simulink model "ENV_scheduled"  (R2024b)
settings: Solver=FixedStepDiscrete  StartTime=0.0  StopTime=10.0  FixedStep=0.001  RelTol=1e-3
libraries: stm32blockslib x54, canmsglib x29, simulink x7, stm32f4xxblockslib x1
(part 1 of 5)
settings Model: DataDictionary=Master_Dictionary.sldd  EnableAccessToBaseWorkspace=off  STM32="{\"SPIControllerTransfer\":[{\"ID\":\"ENV:1198\"},{\"ID\":\"ENV:1199\"},{\"ID\":\"ENV:1337\"},{\"ID\":\"ENV:1338\"},{\"ID\":\"ENV:1339\"},{\"ID\":\"ENV:1340\"},{\"ID\":\"ENV:1341\"},{\"ID\":\"ENV:1354\"},{\"ID\":\"ENV:1361\"},{\"ID\":\"ENV:1368\"},{\"ID\":\"ENV:1375\"},{\"ID\":\"ENV:1394\"},{\"ID\":\"ENV:1413\"},{\"ID\":\"ENV:1469\"},{\"ID\":\"ENV:2306\"},{\"ID\":\"ENV:2307\"},{\"ID\":\"ENV:2328\"},{\"ID\":\"ENV:2329\"},{\"ID\":\"ENV:2371\"},{\"ID\":\"ENV:2372\"},{\"ID\":\"ENV:2383\"},{\"ID\":\"ENV:2384\"},{\"ID\":\"ENV:2395\"},{\"ID\":\"ENV:2396\"},{\"ID\":\"ENV:2407\"},{\"ID\":\"ENV:2408\"},{\"ID\":\"ENV:2419\"},{\"ID\":\"ENV:2420\"},{\"ID\":\"ENV:2431\"},{\"ID\":\"ENV:2432\"},{\"ID\":\"ENV:2443\"},{\"ID\":\"ENV:2444\"},{\"ID\":\"ENV:2455\"},{\"ID\":\"ENV:2456\"},{\"ID\":\"ENV:2467\"},{\"ID\":\"ENV:2468\"},{\"ID\":\"ENV:2479\"},{\"ID\":\"ENV:2480\"},{\"ID\":\"ENV:2491\"},{\"ID\":\"ENV:2492\"},{\"ID\":\"ENV:2503\"},{\"ID\":\"ENV:2504\"},{\"ID\":\"ENV:2515\"},{\"ID\":\"ENV:2516\"},{\"ID\":\"ENV:2527\"},{\"ID\":\"ENV:2528\"},{\"ID\":\"ENV:2539\"},{\"ID\":\"ENV:2540\"},{\"ID\":\"ENV:2551\"},{\"ID\":\"ENV:2552\"},{\"ID\":\"ENV:2563\"},{\"ID\":\"ENV:2564\"},{\"ID\":\"ENV:2575\"},{\"ID\":\"ENV:2576\"}],\"DigitalPortRead\":{\"ID\":\"ENV:1217\"}}"  Creator=oxbro  LastModifiedBy=oxbro
settings SolverCC: AlgebraicLoopSolver=TrustRegion
settings DataIOCC: ReturnWorkspaceOutputs=off
settings OptimizationCC: DefaultParameterBehavior=Inlined  OptimizeBlockIOStorage=off  BufferReuse=off  ReuseModelBlockBuffer=off  GlobalBufferReuse=off  ExpressionFolding=off  EnableMemcpy=off  PassReuseOutputArgsAs=Individual arguments  LocalBlockOutputs=off  ZeroExternalMemoryAtStartup=off  ZeroInternalMemoryAtStartup=off  MaxStackSize=8192  OptimizeDataStoreBuffers=off  BusAssignmentInplaceUpdate=off  OptimizationLevel=level0  OptimizationCustomize=off  EfficientTunableParamExpr=on
settings DebuggingCC: ParameterOverflowMsg=warning  ParameterTunabilityLossMsg=error  UnconnectedInputMsg=warning  UnconnectedOutputMsg=warning  UnconnectedLineMsg=warning  ArithmeticOperatorsInVariantConditions=warning
settings HardwareCC: ProdBitPerPointer=32  ProdBitPerSizeT=32  ProdBitPerPtrDiffT=32  ProdLargestAtomicInteger=Long  ProdLargestAtomicFloat=Double  ProdWordSize=32  ProdLongLongMode=on  ProdHWDeviceType=ARM Compatible->ARM Cortex-M
settings ModelReferenceCC: EnableRefExpFcnMdlSchedulingChecks=on
settings SFSimCC: MATLABDynamicMemAlloc=off  CustomCodeUndefinedFunction=UseInterfaceOnly
settings RTWCC: Description=Embedded Coder  SystemTargetFile=ert.tlc  HardwareBoard=STM32H7xx Based (Single-core)  TemplateMakefile=ert_default_tmf  Toolchain=GNU Tools for ARM Embedded Processors  GPUComputeCapability=3.5
settings CodeAppCC: ForceParamTrailComments=on  IgnoreCustomStorageClasses=off  MaxIdLength=45  OperatorAnnotations=on  SimulinkDataObjDesc=on  SFDataObjDesc=on  InsertBlockDesc=on
settings ERTTargetCC: TargetLangStandard=C99 (ISO)  CodeReplacementLibrary=ARM Cortex-M  ExtModeTransport=3  ExtModeStaticAlloc=on  ExtModeStaticAllocSize=2048  ExtModeMexFile=ext_xcp  ExtModeIntrfLevel=Level2 - Open

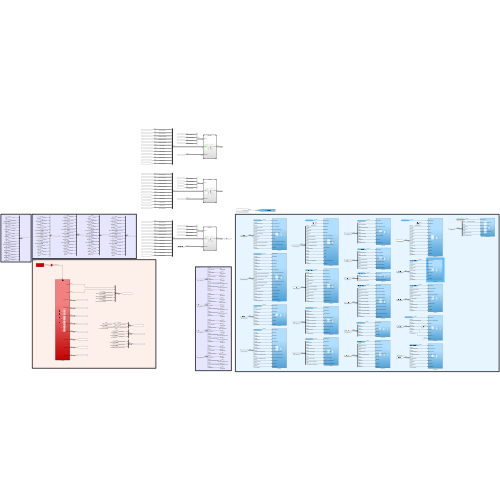
[thumbnail: Simulink's stored preview of the top-level diagram]
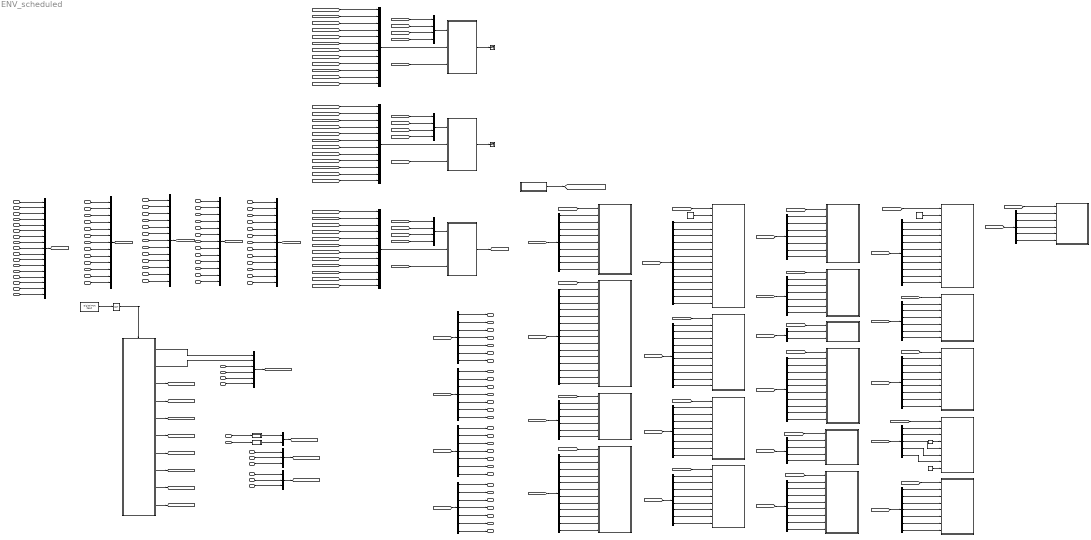
== system ENV_scheduled ==
  note: CAN3
  note: CAN 1&2
  note: CAN3
  note: CAN4
  note: CAN1&2
  nMotorRL : Inport
  BInvDCOnRLIn : Inport  Port=2
  BInvErrorRL : Inport  Port=3
  BInvOnRLIn : Inport  Port=4
  BInvDCQuitInvOnRL : Inport  Port=5
  BInvQuitInvOnRL : Inport  Port=6
  BInvSysReadyRL : Inport  Port=7
  BInvWarnRL : Inport  Port=8
  MMotorMeasuredRL : Inport  Port=9
  NInvDTCRL : Inport  Port=10
  TMotorRL : Inport  Port=11
  VDCInvRL : Inport  Port=12
  TInvRL : Inport  Port=13
  nMotorRR : Inport  Port=14
  BInvDCOnRRIn : Inport  Port=15
  BInvErrorRR : Inport  Port=16
  BInvOnRRIn : Inport  Port=17
  BInvDCQuitInvOnRR : Inport  Port=18
  BInvQuitInvOnRR : Inport  Port=19
  BInvSysReadyRR : Inport  Port=20
  BInvWarnRR : Inport  Port=21
  MMotorMeasuredRR : Inport  Port=22
  NInvDTCRR : Inport  Port=23
  TMotorRR : Inport  Port=24
  VDCInvRR : Inport  Port=25
  TInvRR : Inport  Port=26
  nMotorFL : Inport  Port=27
  BInvDCOnFLIn : Inport  Port=28
  BInvErrorFL : Inport  Port=29
  BInvOnFLIn : Inport  Port=30
  BInvDCQuitInvOnFL : Inport  Port=31
  BInvQuitInvOnFL : Inport  Port=32
  BInvSysReadyFL : Inport  Port=33
  BInvWarnFL : Inport  Port=34
  MMotorMeasuredFL : Inport  Port=35
  NInvDTCFL : Inport  Port=36
  TMotorFL : Inport  Port=37
  VDCInvFL : Inport  Port=38
  TInvFL : Inport  Port=39
  nMotorFR : Inport  Port=40
  BInvDCOnFR : Inport  Port=41
  BInvErrorFR : Inport  Port=42
  BInvOnFR : Inport  Port=43
  BInvDCQuitInvOnFR : Inport  Port=44
  BInvQuitInvOnFR : Inport  Port=45
  BInvSysReadyFR : Inport  Port=46
  BInvWarnFR : Inport  Port=47
  MMotorMeasuredFR : Inport  Port=48
  NInvDTCFR : Inport  Port=49
  TMotorFR : Inport  Port=50
  VDCInvFR : Inport  Port=51
  TInvFR : Inport  Port=52
  IIVTS : Inport  Port=53
  IBMSHallEffect : Inport  Port=54
  VDCAccumulator : Inport  Port=55
  TCellMin : Inport  Port=56
  VCellAverage : Inport  Port=57
  VCellMax : Inport  Port=58
  TCellMax : Inport  Port=59
  NBMSDLC : Inport  Port=60
  VCellMin : Inport  Port=61
  RCellAverage : Inport  Port=62
  BBalancingActive : Inport  Port=63
  BBMSP0A0C : Inport  Port=64  OutDataTypeStr=double
  BBMSP0A0E : Inport  Port=65
  BBMSP0A10 : Inport  Port=66
  BBMSP0A80 : Inport  Port=67
  BBMSP0AC0 : Inport  Port=68
  BBMSP0AFA : Inport  Port=69
  vLateralOXTSIMU : Inport  Port=70
  vLongitudinalOXTSIMU : Inport  Port=71
  gLateralOXTS : Inport  Port=72
  gLongitudinalOXTS : Inport  Port=73
  gVerticalOXTS : Inport  Port=74
  nPitchRateOXTSIMU : Inport  Port=75
  nRollRateOXTSIMU : Inport  Port=76
  nYawRateOXTSIMU : Inport  Port=77
  VDamperPotentiometerFL : Inport  Port=78
  VDamperPotentiometerFR : Inport  Port=79
  VDamperPotentiometerRR : Inport  Port=80
  VDamperPotentiometerRL : Inport  Port=81
  Bus Creator1 : BusCreator  Inputs=6  OutDataTypeStr=Bus: DDU7_Analoge_1
  Bus Creator13 : BusCreator  Inputs=12  OutDataTypeStr=Bus: CAN3Bus
  Bus Creator14 : BusCreator  Inputs=13  OutDataTypeStr=Bus: InverterFLCANBus
  Bus Creator15 : BusCreator  Inputs=13  OutDataTypeStr=Bus: InverterFRCANBus
  Bus Creator16 : BusCreator  Inputs=12  OutDataTypeStr=Bus: CAN3Bus
  Bus Creator17 : BusCreator  Inputs=13  OutDataTypeStr=Bus: InverterRLCANBus
  Bus Creator18 : BusCreator  Inputs=17  OutDataTypeStr=Bus: CAN4Bus
  Bus Creator19 : BusCreator  Inputs=13  OutDataTypeStr=Bus: InverterRRCANBus
  Bus Creator20 : BusCreator  Inputs=12  OutDataTypeStr=Bus: CAN3Bus
  Bus Creator6 : BusCreator  Inputs=3  OutDataTypeStr=Bus: OXTSDataFrame1544
  Bus Creator7 : BusCreator  Inputs=3  OutDataTypeStr=Bus: OXTSDataFrame1541
  Bus Creator8 : BusCreator  Inputs=2  OutDataTypeStr=Bus: OXTSDataFrame1540
  Bus Selector : BusSelector  OutputSignals=SystemsBus.BEncoderErrorFront,SystemsBus.BEncoderErrorRear,SystemsBus.BSpinningModelActivated,TorqueControlBus.BTorqueVectoringOK,TorqueControlBus.MTotalFinal,SystemsBus.PActual,TorqueControlBus.PPowerControllerProportionalTerm,TorqueControlBus.PPowerControllerIntegralTerm,SystemsBus.vChassis
  Bus Selector1 : BusSelector  OutputSignals=BMSSignalsBus.BBMSP0A80,BMSSignalsBus.BBMSP0AC0,BMSSignalsBus.BBMSP0AFA,SystemsBus.PDischarge,LimitationsBus.rDischargeDerate,LimitationsBus.rHighCellTemperatureDischargeDerate,LimitationsBus.rHighCellTemperatureRegenDerate,LimitationsBus.rInvTemperatureDerate,LimitationsBus.rLowCellVoltageDischargeDerate,LimitationsBus.rMotorTemperatureDerate,LimitationsBus.rRegenDerate,LimitationsBus.rSOCDischargeDerate,LimitationsBus.rSOCRegenDerate,TorqueControlBus.rSOCTargetError,LimitationsBus.rSpeedRegenDerate
  Bus Selector10 : BusSelector  OutputSignals=SensorSignalsBus.VDamperPotentiometerFL,SensorSignalsBus.VDamperPotentiometerFR
  Bus Selector11 : BusSelector  OutputSignals=TorqueControlBus.MTotalEMSRequested,LimitationsBus.rInvTemperatureDerateFL,LimitationsBus.rInvTemperatureDerateFR,LimitationsBus.rInvTemperatureDerateRL,LimitationsBus.rInvTemperatureDerateRR,LimitationsBus.rMotorTemperatureDerateFL,LimitationsBus.rMotorTemperatureDerateFR,LimitationsBus.rMotorTemperatureDerateRL,LimitationsBus.rMotorTemperatureDerateRR,SystemsBus.rThrottlePedal
  Bus Selector12 : BusSelector  OutputSignals=InverterSignalsBus.InverterFLSignalsBus.nMotorFL,InverterSignalsBus.InverterFRSignalsBus.nMotorFR,InverterSignalsBus.InverterRLSignalsBus.nMotorRL,InverterSignalsBus.InverterRRSignalsBus.nMotorRR
  Bus Selector13 : BusSelector  OutputSignals=LimitationsBus.BDischargeAllowed,SystemsBus.BEMS1000mPoint,SystemsBus.BEMS995mPoint,TorqueControlBus.MDriverDischargeRequested,TorqueControlBus.MFLFinal,TorqueControlBus.MFRFinal,TorqueControlBus.MRLFinal,TorqueControlBus.MRRFinal
  Bus Selector14 : BusSelector  OutputSignals=InverterSignalsBus.InverterFLSignalsBus.TInvFL,InverterSignalsBus.InverterFRSignalsBus.TInvFR,SystemsBus.TInvMax,InverterSignalsBus.InverterRLSignalsBus.TInvRL,InverterSignalsBus.InverterRRSignalsBus.TInvRR,InverterSignalsBus.InverterFLSignalsBus.TMotorFL,InverterSignalsBus.InverterFRSignalsBus.TMotorFR,SystemsBus.TMotorMax,InverterSignalsBus.InverterRLSignalsBus.TMotorRL,InverterSignalsBus.InverterRRSignalsBus.TMotorRR
  Bus Selector15 : BusSelector  OutputSignals=InverterSignalsBus.InverterFLSignalsBus.NInvDTCFL,InverterSignalsBus.InverterFRSignalsBus.NInvDTCFR,InverterSignalsBus.InverterRLSignalsBus.NInvDTCRL,InverterSignalsBus.InverterRRSignalsBus.NInvDTCRR,BMSSignalsBus.TCellMax,BMSSignalsBus.VCellDelta
  Bus Selector16 : BusSelector  OutputSignals=SystemsBus.BAccumulatorFanOn,SystemsBus.BEMSActivated,SystemsBus.BTractionControlActivated,BMSSignalsBus.IBMSHallEffect,BMSSignalsBus.IIVTS,TorqueControlBus.MTotalRequested,BMSSignalsBus.VDCAccumulator,InverterSignalsBus.InverterRLSignalsBus.VDCInvRL
  Bus Selector17 : BusSelector  OutputSignals=SystemsBus.NTractionControlKpSelector,BMSSignalsBus.TCellMin,BMSSignalsBus.VCellMax,BMSSignalsBus.VCellMin,SensorSignalsBus.VLVSystem
  Bus Selector18 : BusSelector  OutputSignals=TorqueControlBus.PDischargeLimited,SystemsBus.aSteeringAngle,TorqueControlBus.nYawRateErrorActual,SystemsBus.rRegenPaddle,TorqueControlBus.rSplitRear,SystemsBus.tAppsTimer,SystemsBus.tPedalOverlap
  Bus Selector2 : BusSelector  OutputSignals=TorqueControlBus.rSOETargetError,SystemsBus.sEMS1000m,WheelSpeedsBus.vWheelFL,WheelSpeedsBus.vWheelFR,WheelSpeedsBus.vWheelRL,WheelSpeedsBus.vWheelRR
  Bus Selector20 : BusSelector  OutputSignals=StateflowBus.BInvDCOnRL,StateflowBus.BInvEnableRL,StateflowBus.BInvErrorResetRL,StateflowBus.BInvOnRL,StateflowBus.MTorqueLimitNegativeRL,StateflowBus.MTorqueLimitPositiveRL,TorqueControlBus.MRLFinal
  Bus Selector21 : BusSelector  OutputSignals=StateflowBus.BInvDCOnFL,StateflowBus.BInvEnableFL,StateflowBus.BInvErrorResetFL,StateflowBus.BInvOnFL,StateflowBus.MTorqueLimitNegativeFL,StateflowBus.MTorqueLimitPositiveFL,TorqueControlBus.MFLFinal
  Bus Selector22 : BusSelector  OutputSignals=StateflowBus.BInvDCOnRR,StateflowBus.BInvEnableRR,StateflowBus.BInvErrorResetRR,StateflowBus.BInvOnRR,StateflowBus.MTorqueLimitNegativeRR,StateflowBus.MTorqueLimitPositiveRR,TorqueControlBus.MRRFinal
  Bus Selector23 : BusSelector  OutputSignals=StateflowBus.BInvDCOnFR,StateflowBus.BInvEnableFR,StateflowBus.BInvErrorResetFR,StateflowBus.BInvOnFR,StateflowBus.MTorqueLimitNegativeFR,StateflowBus.MTorqueLimitPositiveFR,TorqueControlBus.MFRFinal
  Bus Selector27 : BusSelector  OutputSignals=SystemsBus.BAccumulatorFanOn,SystemsBus.BBrakeLight,SystemsBus.BInvLVOn,StateflowBus.BReadyToDriveBuzzer,SystemsBus.BAccumulatorFanDuty
  Bus Selector3 : BusSelector  OutputSignals=SystemsBus.BAppsOK,SystemsBus.BBrakeError,SystemsBus.BBrakeOn,SystemsBus.BPedalOverlap,SystemsBus.BRegenOn,SystemsBus.BThrottleError,SystemsBus.BTorqueVectoringActivated,TorqueControlBus.MPowerControllerRequested,TorqueControlBus.PPowerControllerRequested,SystemsBus.rThrottlePedal,SystemsBus.tBrakeError,SystemsBus.tThrottleError
  Bus Selector4 : BusSelector  OutputSignals=StateflowBus.BReadyToDrive,TorqueControlBus.NABSMultiplierRL,TorqueControlBus.NABSMultiplierRR,SystemsBus.NThrottleMap,TorqueControlBus.NTractionControlMultiplierRL,TorqueControlBus.NTractionControlMultiplierRR,TorqueControlBus.rSlipRatioFLActual,TorqueControlBus.rSlipRatioFRActual,TorqueControlBus.rSlipRatioRLActual,TorqueControlBus.rSlipRatioRRActual
  Bus Selector5 : BusSelector  OutputSignals=BMSSignalsBus.NBMSDLC,StateflowBus.NBMSState,StateflowBus.NInvState,SystemsBus.NModeNumberDisplay5,SystemsBus.NModeNumberDisplay6,SystemsBus.NPowerControllerKpSelector,SystemsBus.NTorqueSplitSpeedSelector,SystemsBus.PEngineBraking,SystemsBus.PRegen,SystemsBus.rSOC,SystemsBus.rSOE,SystemsBus.rTorqueVectoringMultiplier,SystemsBus.sChassis
  Bus Selector6 : BusSelector  OutputSignals=BMSSignalsBus.BBMSP0A0C,BMSSignalsBus.BBalancingActive,TorqueControlBus.MTractionControlFLTotal,TorqueControlBus.MTractionControlFRTotal,TorqueControlBus.MTractionControlRLTotal,TorqueControlBus.MTractionControlRRTotal,TorqueControlBus.NABSMultiplierFL,TorqueControlBus.NABSMultiplierFR
  Bus Selector7 : BusSelector  OutputSignals=BMSSignalsBus.BBMSP0A0E,BMSSignalsBus.BBMSP0A10,TorqueControlBus.MTorqueVectoringFL,TorqueControlBus.MTorqueVectoringFR,TorqueControlBus.MTorqueVectoringRL,TorqueControlBus.MTorqueVectoringRR,TorqueControlBus.NTractionControlMultiplierFL,TorqueControlBus.NTractionControlMultiplierFR
  Bus Selector8 : BusSelector  OutputSignals=TorqueControlBus.MDischargeLimited,TorqueControlBus.MDriverRegenRequested,TorqueControlBus.MRegenLimited,TorqueControlBus.MSpinningModelFL,TorqueControlBus.MSpinningModelFR,StateflowBus.NCarState,TorqueControlBus.rSlipRatioOptimal
  Bus Selector9 : BusSelector  OutputSignals=TorqueControlBus.MSpinningModelRL,TorqueControlBus.MSpinningModelRR,TorqueControlBus.MTorqueDistributionFL,TorqueControlBus.MTorqueDistributionFR,TorqueControlBus.MTorqueDistributionRL,TorqueControlBus.MTorqueDistributionRR
  CAN Rx : Subsystem  TreatAsAtomicUnit=on
  CAN Tx : Subsystem
  CAN Tx1 : Subsystem
  CAN Tx10 : Subsystem
  CAN Tx11 : Subsystem
  CAN Tx12 : Subsystem
  CAN Tx13 : Subsystem
  CAN Tx14 : Subsystem
  CAN Tx15 : Subsystem
  CAN Tx16 : Subsystem
  CAN Tx17 : Subsystem
  CAN Tx18 : Subsystem
  CAN Tx19 : Subsystem
  CAN Tx2 : Subsystem
  CAN Tx3 : Subsystem
  CAN Tx4 : Subsystem
  CAN Tx5 : Subsystem
  CAN Tx6 : Subsystem
  CAN Tx7 : Subsystem
  CAN Tx8 : Subsystem
  CAN Tx9 : Subsystem
  CAN1_2Bus : BusCreator  Inputs=4  OutDataTypeStr=Bus: CAN1_2Bus
  CAN1_2Bus1 : BusCreator  Inputs=4  OutDataTypeStr=Bus: CAN1_2Bus
  CAN1_2Bus2 : BusCreator  Inputs=4  OutDataTypeStr=Bus: CAN1_2Bus
  Constant : Constant  Value=92
  Constant1 : Constant  Value=92
  Digital Port Read1 : stm32f4xxblockslib/Digital Port Read  PortName=GPIOB  PinNumber=5  ReadOperation=on  IOAsArray=off  SampleTime=-1  EnableSimPort=off  hoistedMaskSrc=ECSoC/ECSimCodegen/Digital Port Read
      settings: LibrarySourceBlock=stm32f2xxblockslib/Digital Port Read
  Model : ModelReference  ModelNameDialog=MASTER.slx  SimulationMode=Normal  ModelReferenceVersion=13.13
  Model1 : ModelReference  ModelNameDialog=MASTER.slx  SimulationMode=Normal  ModelReferenceVersion=13.13
  Model2 : ModelReference  ModelNameDialog=MASTER.slx  SimulationMode=Normal  ModelReferenceVersion=13.13
  Multiplexer1? : simulink/Sources/Counter Limited  uplimit=1  tsamp=5
  Multiplexer? : simulink/Sources/Counter Limited  uplimit=1  tsamp=5
  NOT4 : Logic  Operator=NOT  IconShape=distinctive  AllPortsSameDT=off  OutDataTypeStr=boolean
  Subsystem : Subsystem
  Terminator : Terminator
  Terminator1 : Terminator
  gLat : Subsystem
  gLong : Subsystem
  BInvDCOnRL : Outport  VectorParamsAs1DForOutWhenUnconnected=off
  BInvEnableRL : Outport  Port=2  VectorParamsAs1DForOutWhenUnconnected=off
  BInvErrorResetRL : Outport  Port=3  VectorParamsAs1DForOutWhenUnconnected=off
  BInvOnRL : Outport  Port=4  VectorParamsAs1DForOutWhenUnconnected=off
  MTorqueLimitNegativeRL : Outport  Port=5  VectorParamsAs1DForOutWhenUnconnected=off
  MTorqueLimitPositiveRL : Outport  Port=6  VectorParamsAs1DForOutWhenUnconnected=off
  MInvRLFinal : Outport  Port=7  VectorParamsAs1DForOutWhenUnconnected=off
  BInvDCOnFL : Outport  Port=8  VectorParamsAs1DForOutWhenUnconnected=off
  BInvEnableFL : Outport  Port=9  VectorParamsAs1DForOutWhenUnconnected=off
  BInvErrorResetFL : Outport  Port=10  VectorParamsAs1DForOutWhenUnconnected=off
  BInvOnFL : Outport  Port=11  VectorParamsAs1DForOutWhenUnconnected=off
  MTorqueLimitNegativeFL : Outport  Port=12  VectorParamsAs1DForOutWhenUnconnected=off
  MTorqueLimitPositiveFL : Outport  Port=13  VectorParamsAs1DForOutWhenUnconnected=off
  MInvFLFinal : Outport  Port=14  VectorParamsAs1DForOutWhenUnconnected=off
  BInvDCOnRR : Outport  Port=15  VectorParamsAs1DForOutWhenUnconnected=off
  BInvEnableRR : Outport  Port=16  VectorParamsAs1DForOutWhenUnconnected=off
  BInvErrorResetRR : Outport  Port=17  VectorParamsAs1DForOutWhenUnconnected=off
  BInvOnRR : Outport  Port=18  VectorParamsAs1DForOutWhenUnconnected=off
  MTorqueLimitNegativeRR : Outport  Port=19  VectorParamsAs1DForOutWhenUnconnected=off
  MTorqueLimitPositiveRR : Outport  Port=20  VectorParamsAs1DForOutWhenUnconnected=off
  MInvRRFinal : Outport  Port=21  VectorParamsAs1DForOutWhenUnconnected=off
  "BInvDCOnFR " : Outport  Port=22  VectorParamsAs1DForOutWhenUnconnected=off
  BInvEnableFR : Outport  Port=23  VectorParamsAs1DForOutWhenUnconnected=off
  BInvErrorResetFR : Outport  Port=24  VectorParamsAs1DForOutWhenUnconnected=off
  "BInvOnFR " : Outport  Port=25  VectorParamsAs1DForOutWhenUnconnected=off
  MTorqueLimitNegativeFR : Outport  Port=26  VectorParamsAs1DForOutWhenUnconnected=off
  MTorqueLimitPositiveFR : Outport  Port=27  VectorParamsAs1DForOutWhenUnconnected=off
  MInvFRFinal : Outport  Port=28  VectorParamsAs1DForOutWhenUnconnected=off
  wires:
  nMotorRL/1 -> Bus Creator17/1  "nMotorRL"
  BInvDCOnRLIn/1 -> Bus Creator17/2  "BInvDCOnRL"
  BInvErrorRL/1 -> Bus Creator17/3  "BInvErrorRL"
  BInvOnRLIn/1 -> Bus Creator17/4  "BInvOnRL"
  BInvDCQuitInvOnRL/1 -> Bus Creator17/5  "BInvDCQuitInvOnRL"
  BInvSysReadyRL/1 -> Bus Creator17/7  "BInvSysReadyRL"
  BInvWarnRL/1 -> Bus Creator17/8  "BInvWarnRL"
  MMotorMeasuredRL/1 -> Bus Creator17/9  "MMotorMeasuredRL"
  NInvDTCRL/1 -> Bus Creator17/10  "NInvDTCRL"
  TMotorRL/1 -> Bus Creator17/11  "TMotorRL"
  VDCInvRL/1 -> Bus Creator17/12  "VDCInvRL"
  MMotorMeasuredRR/1 -> Bus Creator19/9  "MMotorMeasuredRR"
  BInvSysReadyRR/1 -> Bus Creator19/7  "BInvSysReadyRR"
  TMotorRR/1 -> Bus Creator19/11  "TMotorRR"
  BInvErrorRR/1 -> Bus Creator19/3  "BInvErrorRR"
  nMotorRR/1 -> Bus Creator19/1  "nMotorRR"
  BInvDCQuitInvOnRR/1 -> Bus Creator19/5  "BInvDCQuitInvOnRR"
  BInvDCOnRRIn/1 -> Bus Creator19/2  "BInvDCOnRR"
  BInvWarnRR/1 -> Bus Creator19/8  "BInvWarnRR"
  NInvDTCRR/1 -> Bus Creator19/10  "NInvDTCRR"
  VDCInvRR/1 -> Bus Creator19/12  "VDCInvRR"
  BInvOnRRIn/1 -> Bus Creator19/4  "BInvOnRR"
  BInvOnFLIn/1 -> Bus Creator14/4  "BInvOnFL"
  VDCInvFL/1 -> Bus Creator14/12  "VDCInvFL"
  BInvWarnFL/1 -> Bus Creator14/8  "BInvWarnFL"
  BInvDCQuitInvOnFL/1 -> Bus Creator14/5  "BInvDCQuitInvOnFL"
  NInvDTCFL/1 -> Bus Creator14/10  "NInvDTCFL"
  BInvErrorFL/1 -> Bus Creator14/3  "BInvErrorFL"
  BInvDCOnFLIn/1 -> Bus Creator14/2  "BInvDCOnFL"
  TMotorFL/1 -> Bus Creator14/11  "TMotorFL"
  nMotorFL/1 -> Bus Creator14/1  "nMotorFL"
  BInvSysReadyFL/1 -> Bus Creator14/7  "BInvSysReadyFL"
  MMotorMeasuredFL/1 -> Bus Creator14/9  "MMotorMeasuredFL"
  BInvDCOnFR/1 -> Bus Creator15/2  "BInvDCOnFR"
  BInvErrorFR/1 -> Bus Creator15/3  "BInvErrorFR"
  MMotorMeasuredFR/1 -> Bus Creator15/9  "MMotorMeasuredFR"
  BInvSysReadyFR/1 -> Bus Creator15/7  "BInvSysReadyFR"
  nMotorFR/1 -> Bus Creator15/1  "nMotorFR"
  TMotorFR/1 -> Bus Creator15/11  "TMotorFR"
  NInvDTCFR/1 -> Bus Creator15/10  "NInvDTCFR"
  VDCInvFR/1 -> Bus Creator15/12  "VDCInvFR"
  BInvDCQuitInvOnFR/1 -> Bus Creator15/5  "BInvDCQuitInvOnFR"
  BInvWarnFR/1 -> Bus Creator15/8  "BInvWarnFR"
  BInvOnFR/1 -> Bus Creator15/4  "BInvOnFR"
  Bus Creator17/1 -> [InverterRLBus]
  Bus Creator14/1 -> [InverterFLBus]
  Bus Creator15/1 -> [InverterFRBus]
  IIVTS/1 -> Bus Creator18/1  "IIVTS"
  TCellMin/1 -> Bus Creator18/4  "TCellMin"
  RCellAverage/1 -> Bus Creator18/10  "RCellAverage"
  TCellMax/1 -> Bus Creator18/7  "TCellMax"
  BBMSP0A80/1 -> Bus Creator18/15  "BBMSP0A80"
  IBMSHallEffect/1 -> Bus Creator18/2  "IBMSHallEffect"
  VDCAccumulator/1 -> Bus Creator18/3  "VDCAccumulator"
  VCellAverage/1 -> Bus Creator18/5  "VCellAverage"
  NBMSDLC/1 -> Bus Creator18/8  "NBMSDLC"
  VCellMin/1 -> Bus Creator18/9  "VCellMin"
  VCellMax/1 -> Bus Creator18/6  "VCellMax"
  BBalancingActive/1 -> Bus Creator18/11  "BBalancingActive"
  BBMSP0A0C/1 -> Bus Creator18/12  "BBMSP0A0C"
  BBMSP0A0E/1 -> Bus Creator18/13  "BBMSP0A0E"
  BBMSP0A10/1 -> Bus Creator18/14  "BBMSP0A10"
  BBMSP0AC0/1 -> Bus Creator18/16  "BBMSP0AC0"
  BBMSP0AFA/1 -> Bus Creator18/17  "BBMSP0AFA"
  Bus Creator18/1 -> [BMSCAN]
  Bus Creator1/1 -> [DDU7_Analoge_1]
  Bus Creator8/1 -> [OXTSDataFrame1540]
  gLateralOXTS/1 -> Bus Creator7/1  "gLateralOXTS"
  gLongitudinalOXTS/1 -> Bus Creator7/2  "gLongitudinalOXTS"
  gVerticalOXTS/1 -> Bus Creator7/3  "gVerticalOXTS"
  Bus Creator7/1 -> [OXTSDataFrame1541]
  nPitchRateOXTSIMU/1 -> Bus Creator6/1  "nPitchRateOXTSIMU"
  nRollRateOXTSIMU/1 -> Bus Creator6/2  "nRollRateOXTSIMU"
  nYawRateOXTSIMU/1 -> Bus Creator6/3  "nYawRateOXTSIMU"
  Bus Creator6/1 -> [OXTSDataFrame1544]
  CAN1_2Bus/1 -> Model/1
  [BMSCAN] -> Model/3
  [DDU7_Analoge_1] -> Bus Creator13/1  "DDU7_Analoge_1"
  [DDU7_Analoge_2] -> Bus Creator13/2  "DDU7_Analoge_2"
  [OXTSDataFrame1540] -> Bus Creator13/3  "OXTSDataFrame1540"
  [OXTSDataFrame1541] -> Bus Creator13/4  "OXTSDataFrame1541"
  [OXTSDataFrame1544] -> Bus Creator13/5  "OXTSDataFrame1544"
  [PDM_Status_1] -> Bus Creator13/6  "PDM_Status_1"
  [PDM_Status_2] -> Bus Creator13/7  "PDM_Status_2"
  [PDM_Status_3] -> Bus Creator13/8  "PDM_Status_3"
  [PDM_Analog_1] -> Bus Creator13/9  "PDM_Analoge_1"
  [PDM_Analoge_2] -> Bus Creator13/10  "PDM_Analoge_2"
  [PDM_Analoge_3] -> Bus Creator13/11  "PDM_Analoge_3"
  [SteeringWheelBus] -> Bus Creator13/12  "SteeringWheelBus"
  Bus Creator13/1 -> Model/2
  Model/1 -> [Global]
  TInvRL/1 -> Bus Creator17/13  "TInvRL"
  TInvRR/1 -> Bus Creator19/13  "TInvRR"
  TInvFL/1 -> Bus Creator14/13  "TInvFL"
  TInvFR/1 -> Bus Creator15/13  "TInvFR"
  BInvQuitInvOnRL/1 -> Bus Creator17/6  "BInvQuitInvOnRL"
  BInvQuitInvOnRR/1 -> Bus Creator19/6  "BInvQuitInvOnRR"
  BInvQuitInvOnFL/1 -> Bus Creator14/6  "BInvQuitInvOnFL"
  BInvQuitInvOnFR/1 -> Bus Creator15/6  "BInvQuitInvOnFR"
  [Global] -> Bus Selector/1
  [Global] -> Bus Selector1/1
  [Global] -> Bus Selector2/1
  [Global] -> Bus Selector3/1
  [Global] -> Bus Selector4/1
  [Global] -> Bus Selector5/1
  [Global] -> Bus Selector6/1
  [Global] -> Bus Selector7/1
  [Global] -> Bus Selector8/1
  [Global] -> Bus Selector9/1
  [Global] -> Bus Selector10/1
  [Global] -> Bus Selector11/1
  [Global] -> Bus Selector12/1
  [Global] -> Bus Selector13/1
  [Global] -> Bus Selector14/1
  [Global] -> Bus Selector15/1
  [Global] -> Bus Selector16/1
  [Global] -> Bus Selector17/1
  [Global] -> Bus Selector18/1
  [Global] -> Bus Selector20/1
  Bus Selector20/1 -> BInvDCOnRL/1  "<BInvDCOnRL>"
  Bus Selector20/2 -> BInvEnableRL/1  "<BInvEnableRL>"
  Bus Selector20/3 -> BInvErrorResetRL/1  "<BInvErrorResetRL>"
  Bus Selector20/4 -> BInvOnRL/1  "<BInvOnRL>"
  Bus Selector20/5 -> MTorqueLimitNegativeRL/1  "<MTorqueLimitNegativeRL>"
  Bus Selector20/6 -> MTorqueLimitPositiveRL/1  "<MTorqueLimitPositiveRL>"
  Bus Selector20/7 -> MInvRLFinal/1  "<MRLFinal>"
  [Global] -> Bus Selector21/1
  Bus Selector21/5 -> MTorqueLimitNegativeFL/1  "<MTorqueLimitNegativeFL>"
  Bus Selector21/2 -> BInvEnableFL/1  "<BInvEnableFL>"
  Bus Selector21/7 -> MInvFLFinal/1  "<MFLFinal>"
  Bus Selector21/6 -> MTorqueLimitPositiveFL/1  "<MTorqueLimitPositiveFL>"
  Bus Selector21/3 -> BInvErrorResetFL/1  "<BInvErrorResetFL>"
  Bus Selector21/1 -> BInvDCOnFL/1  "<BInvDCOnFL>"
  Bus Selector21/4 -> BInvOnFL/1  "<BInvOnFL>"
  Bus Selector22/4 -> BInvOnRR/1  "<BInvOnRR>"
  Bus Selector22/6 -> MTorqueLimitPositiveRR/1  "<MTorqueLimitPositiveRR>"
  Bus Selector22/7 -> MInvRRFinal/1  "<MRRFinal>"
  Bus Selector22/3 -> BInvErrorResetRR/1  "<BInvErrorResetRR>"
  Bus Selector22/1 -> BInvDCOnRR/1  "<BInvDCOnRR>"
  [Global] -> Bus Selector22/1
  Bus Selector22/2 -> BInvEnableRR/1  "<BInvEnableRR>"
  Bus Selector22/5 -> MTorqueLimitNegativeRR/1  "<MTorqueLimitNegativeRR>"
  Bus Selector23/2 -> BInvEnableFR/1  "<BInvEnableFR>"
  Bus Selector23/5 -> MTorqueLimitNegativeFR/1  "<MTorqueLimitNegativeFR>"
  Bus Selector23/1 -> "BInvDCOnFR "/1  "<BInvDCOnFR>"
  [Global] -> Bus Selector23/1
  Bus Selector23/3 -> BInvErrorResetFR/1  "<BInvErrorResetFR>"
  Bus Selector23/6 -> MTorqueLimitPositiveFR/1  "<MTorqueLimitPositiveFR>"
  Bus Selector23/4 -> "BInvOnFR "/1  "<BInvOnFR>"
  Bus Selector23/7 -> MInvFRFinal/1  "<MFRFinal>"
  VDamperPotentiometerFL/1 -> Bus Creator1/3  "VDamperPotentiometerFL"
  VDamperPotentiometerFR/1 -> Bus Creator1/4  "VDamperPotentiometerFR"
  [Global] -> Bus Selector27/1
  Bus Selector27/1 -> CAN Tx19/2(BAccumulatorFanOnRequest)  "<BAccumulatorFanOn>"
  Bus Selector27/3 -> CAN Tx19/4(BInvLVOnRequest)  "<BInvLVOn>"
  Bus Selector27/4 -> CAN Tx19/5(BReadyToDriveBuzzerRequest)  "<BReadyToDriveBuzzer>"
  Bus Selector27/5 -> CAN Tx19/6(Other)  "<BAccumulatorFanDuty>"
  Bus Selector27/2 -> CAN Tx19/3(BBrakeLightOnRequest)  "<BBrakeLight>"
  vLateralOXTSIMU/1 -> gLat/1(In1)  "vLateralOXTSIMU"
  gLat/1(Out1) -> Bus Creator8/1  "vLateralOXTSIMU"
  vLongitudinalOXTSIMU/1 -> gLong/1(In1)  "vLongitudinalOXTSIMU"
  gLong/1(Out1) -> Bus Creator8/2  "vLongitudinalOXTSIMU"
  Bus Selector/7 -> CAN Tx/8(PPowerControllerProportionalTerm)  "<PPowerControllerProportionalTerm>"
  Bus Selector/8 -> CAN Tx/9(PPowerControllerIntegralTerm)  "<PPowerControllerIntegralTerm>"
  Bus Selector/6 -> CAN Tx/7(PActual)  "<PActual>"
  Bus Selector/5 -> CAN Tx/6(MTotalFinal)  "<MTotalFinal>"
  Bus Selector/9 -> CAN Tx/10(VChassis)  "<vChassis>"
  Bus Selector/3 -> CAN Tx/4(BSpinningModelActivated)  "<BSpinningModelActivated>"
  Bus Selector/4 -> CAN Tx/5(BTorqueVectoringOk)  "<BTorqueVectoringOK>"
  Bus Selector/2 -> CAN Tx/3(BEncoderErrorRear)  "<BEncoderErrorRear>"
  Bus Selector/1 -> CAN Tx/2(BEncoderErrorFront)  "<BEncoderErrorFront>"
  Bus Selector1/1 -> CAN Tx1/2(BBMSP0A80)  "<BBMSP0A80>"
  Bus Selector1/2 -> CAN Tx1/3(BBMSP0AC0)  "<BBMSP0AC0>"
  Bus Selector1/3 -> CAN Tx1/4(BBMSP0AFA)  "<BBMSP0AFA>"
  Bus Selector1/6 -> CAN Tx1/7(rHighCellTempDischargeDerate)  "<rHighCellTemperatureDischargeDerate>"
  Bus Selector1/7 -> CAN Tx1/8(rHighCellTempRegenDerate)  "<rHighCellTemperatureRegenDerate>"
  Bus Selector1/8 -> CAN Tx1/9(rInvTemperatureDerate)  "<rInvTemperatureDerate>"
  Bus Selector1/10 -> CAN Tx1/11(rMotorTemperatureDerate)  "<rMotorTemperatureDerate>"
  Bus Selector1/9 -> CAN Tx1/10(rLowCellVoltageDischargeDerate)  "<rLowCellVoltageDischargeDerate>"
  Bus Selector1/12 -> CAN Tx1/13(rSOCDischargeDerate)  "<rSOCDischargeDerate>"
  Bus Selector1/13 -> CAN Tx1/14(rSOCRegenDerate)  "<rSOCRegenDerate>"
  Bus Selector1/15 -> CAN Tx1/16(rSpeedRegenDerate)  "<rSpeedRegenDerate>"
  Bus Selector1/5 -> CAN Tx1/6(rDischargeDerate)  "<rDischargeDerate>"
  Bus Selector1/11 -> CAN Tx1/12(rRegenDerate)  "<rRegenDerate>"
  Bus Selector1/4 -> CAN Tx1/5(PDischarge)  "<PDischarge>"
  Bus Selector1/14 -> CAN Tx1/15(rSOCTargetError)  "<rSOCTargetError>"
  Bus Selector2/2 -> CAN Tx2/3(sEMS1000m)  "<sEMS1000m>"
  Bus Selector2/5 -> CAN Tx2/6(vWheelRL)  "<vWheelRL>"
  Bus Selector2/6 -> CAN Tx2/7(vWheelRR)  "<vWheelRR>"
  Bus Selector2/3 -> CAN Tx2/4(vWheelFL)  "<vWheelFL>"
  Bus Selector2/4 -> CAN Tx2/5(vWheelFR)  "<vWheelFR>"
  Bus Selector3/9 -> CAN Tx3/10(PPowerControllerRequested)  "<PPowerControllerRequested>"
  Bus Selector3/8 -> CAN Tx3/9(MPowerControllerRequested)  "<MPowerControllerRequested>"
  Bus Selector3/10 -> CAN Tx3/11(rThrottlePedal)  "<rThrottlePedal>"
  Bus Selector3/6 -> CAN Tx3/7(BThrottleError)  "<BThrottleError>"
  Bus Selector3/12 -> CAN Tx3/13(tThrottleError)  "<tThrottleError>"
  Bus Selector3/2 -> CAN Tx3/3(BBrakeError)  "<BBrakeError>"
  Bus Selector3/11 -> CAN Tx3/12(tBrakeError)  "<tBrakeError>"
  Bus Selector3/3 -> CAN Tx3/4(BBrakeOn)  "<BBrakeOn>"
  Bus Selector3/4 -> CAN Tx3/5(BPedalOverlap)  "<BPedalOverlap>"
  Bus Selector3/1 -> CAN Tx3/2(BAppsOk)  "<BAppsOK>"
  Bus Selector3/5 -> CAN Tx3/6(BRegenOn)  "<BRegenOn>"
  Bus Selector3/7 -> CAN Tx3/8(BTorqueVectoringActivated)  "<BTorqueVectoringActivated>"
  Bus Selector5/11 -> CAN Tx4/13(rSOE)  "<rSOE>"
  Bus Selector5/13 -> CAN Tx4/15(sChassis)  "<sChassis>"
  Bus Selector5/9 -> CAN Tx4/11(PRegen)  "<PRegen>"
  Bus Selector5/12 -> CAN Tx4/14(rTorqueVectoringMultiplier)  "<rTorqueVectoringMultiplier>"
  Bus Selector5/4 -> CAN Tx4/6(NModeNumberDisplay5)  "<NModeNumberDisplay5>"
  Bus Selector5/8 -> CAN Tx4/10(PEngineBraking)  "<PEngineBraking>"
  Bus Selector5/5 -> CAN Tx4/7(NModeNumberDisplay6)  "<NModeNumberDisplay6>"
  Bus Selector5/6 -> CAN Tx4/8(NPowerControllerKpSelector)  "<NPowerControllerKpSelector>"
  Bus Selector5/7 -> CAN Tx4/9(NTorqueSplitSpeedSelector)  "<NTorqueSplitSpeedSelector>"
  Bus Selector5/1 -> CAN Tx4/3(NBMSDLC)  "<NBMSDLC>"
  Bus Selector5/3 -> CAN Tx4/5(NInvState)  "<NInvState>"
  Bus Selector4/7 -> CAN Tx5/8(rSlipRatioFLActual)  "<rSlipRatioFLActual>"
  Bus Selector4/8 -> CAN Tx5/9(rSlipRatioFRActual)  "<rSlipRatioFRActual>"
  Bus Selector4/9 -> CAN Tx5/10(rSlipRatioRLActual)  "<rSlipRatioRLActual>"
  Bus Selector4/10 -> CAN Tx5/11(rSlipRatioRRActual)  "<rSlipRatioRRActual>"
  Bus Selector4/6 -> CAN Tx5/7(NTractionControlMultiplierRR)  "<NTractionControlMultiplierRR>"
  Bus Selector4/3 -> CAN Tx5/4(NABSMultiplierRR)  "<NABSMultiplierRR>"
  Bus Selector4/5 -> CAN Tx5/6(NTractionControlMultiplierRL)  "<NTractionControlMultiplierRL>"
  Bus Selector4/2 -> CAN Tx5/3(NABSMultiplierRL)  "<NABSMultiplierRL>"
  Bus Selector4/4 -> CAN Tx5/5(NThrottleMap)  "<NThrottleMap>"
  Bus Selector4/1 -> CAN Tx5/2(BReadyToDrive)  "<BReadyToDrive>"
  Bus Selector6/4 -> CAN Tx6/5(MTractionControlFRTotal)  "<MTractionControlFRTotal>"
  Bus Selector6/6 -> CAN Tx6/7(MTractionControlRRTotal)  "<MTractionControlRRTotal>"
  Bus Selector6/5 -> CAN Tx6/6(MTractionControlRLTotal)  "<MTractionControlRLTotal>"
  Bus Selector6/3 -> CAN Tx6/4(MTractionControlFLTotal)  "<MTractionControlFLTotal>"
  Bus Selector6/7 -> CAN Tx6/8(NABSMultiplierFL)  "<NABSMultiplierFL>"
  Bus Selector6/8 -> CAN Tx6/9(NABSMultiplierFR)  "<NABSMultiplierFR>"
  Bus Selector6/2 -> CAN Tx6/3(BBalancingActive)  "<BBalancingActive>"
  Bus Selector6/1 -> CAN Tx6/2(BBMSP0A0C)  "<BBMSP0A0C>"
  Bus Selector7/3 -> CAN Tx7/4(MTorqueVectoringFL)  "<MTorqueVectoringFL>"
  Bus Selector7/4 -> CAN Tx7/5(MTorqueVectoringFR)  "<MTorqueVectoringFR>"
  Bus Selector7/5 -> CAN Tx7/6(MTorqueVectoringRL)  "<MTorqueVectoringRL>"
  Bus Selector7/6 -> CAN Tx7/7(MTorqueVectoringRR)  "<MTorqueVectoringRR>"
  Bus Selector7/7 -> CAN Tx7/8(NTractionControlMultiplierFL)  "<NTractionControlMultiplierFL>"
  Bus Selector7/8 -> CAN Tx7/9(NTractionControlMultiplierFR)  "<NTractionControlMultiplierFR>"
  Bus Selector7/1 -> CAN Tx7/2(BBMSP0A0E)  "<BBMSP0A0E>"
  Bus Selector7/2 -> CAN Tx7/3(BBMSP0A10)  "<BBMSP0A10>"
  Bus Selector8/1 -> CAN Tx8/2(MDischargeLimited)  "<MDischargeLimited>"
  Bus Selector8/2 -> CAN Tx8/3(MDriverRegenRequested)  "<MDriverRegenRequested>"
  Bus Selector8/7 -> CAN Tx8/8(rSlipRatioOptimal)  "<rSlipRatioOptimal>"
  Bus Selector8/3 -> CAN Tx8/4(MRegenLimited)  "<MRegenLimited>"
  Bus Selector8/4 -> CAN Tx8/5(MSpinningModelFL)  "<MSpinningModelFL>"
  Bus Selector8/5 -> CAN Tx8/6(MSpinningModelFR)  "<MSpinningModelFR>"
  Bus Selector8/6 -> CAN Tx8/7(NCarState)  "<NCarState>"
  Bus Selector9/1 -> CAN Tx9/2(MSpinningModelRL)  "<MSpinningModelRL>"
  Bus Selector9/2 -> CAN Tx9/3(MSpinningModelRR)  "<MSpinningModelRR>"
  Bus Selector9/3 -> CAN Tx9/4(MTorqueDistributionFL)  "<MTorqueDistributionFL>"
  Bus Selector9/4 -> CAN Tx9/5(MTorqueDistributionFR)  "<MTorqueDistributionFR>"
  Bus Selector9/5 -> CAN Tx9/6(MTorqueDistributionRL)  "<MTorqueDistributionRL>"
  Bus Selector9/6 -> CAN Tx9/7(MTorqueDistributionRR)  "<MTorqueDistributionRR>"
  Bus Selector10/1 -> CAN Tx10/2(VDamperPotentiometerRL)  "<VDamperPotentiometerFL>"
  Bus Selector10/2 -> CAN Tx10/3(VDamperPotentiometerRR)  "<VDamperPotentiometerFR>"
  Bus Selector11/7 -> CAN Tx11/8(rMotorTemperatureDerateFR)  "<rMotorTemperatureDerateFR>"
  Bus Selector11/6 -> CAN Tx11/7(rMotorTemperatureDerateFL)  "<rMotorTemperatureDerateFL>"
  Bus Selector11/9 -> CAN Tx11/10(rMotorTemperatureDerateRR)  "<rMotorTemperatureDerateRR>"
  Bus Selector11/8 -> CAN Tx11/9(rMotorTemperatureDerateRL)  "<rMotorTemperatureDerateRL>"
  Bus Selector11/3 -> CAN Tx11/4(rInvTemperatureDerateFR)  "<rInvTemperatureDerateFR>"
  Bus Selector11/2 -> CAN Tx11/3(rInvTemperatureDerateFL)  "<rInvTemperatureDerateFL>"
  Bus Selector11/5 -> CAN Tx11/6(rInvTemperatureDerateRR)  "<rInvTemperatureDerateRR>"
  Bus Selector11/4 -> CAN Tx11/5(rInvTemperatureDerateRL)  "<rInvTemperatureDerateRL>"
  Bus Selector11/1 -> CAN Tx11/2(MTotalEMSRequested)  "<MTotalEMSRequested>"
  Bus Selector11/10 -> CAN Tx11/11(rThrottlePedal1)  "<rThrottlePedal>"
  Bus Selector12/3 -> CAN Tx12/4(nMotorRL)  "<nMotorRL>"
  Bus Selector12/1 -> CAN Tx12/2(nMotorFL)  "<nMotorFL>"
  Bus Selector12/4 -> CAN Tx12/5(nMotorRR)  "<nMotorRR>"
  Bus Selector12/2 -> CAN Tx12/3(nMotorFR)  "<nMotorFR>"
  Bus Selector13/5 -> CAN Tx13/6(MFLFinal)  "<MFLFinal>"
  Bus Selector13/6 -> CAN Tx13/7(MFRFinal)  "<MFRFinal>"
  Bus Selector13/7 -> CAN Tx13/8(MRLFinal)  "<MRLFinal>"
  Bus Selector13/8 -> CAN Tx13/9(MRRFinal)  "<MRRFinal>"
  Bus Selector13/4 -> CAN Tx13/5(MDriverDischargeRequested)  "<MDriverDischargeRequested>"
  Bus Selector13/2 -> CAN Tx13/3(BEMS1000mPoint)  "<BEMS1000mPoint>"
  Bus Selector13/3 -> CAN Tx13/4(BEMS995mPoint)  "<BEMS995mPoint>"
  Bus Selector13/1 -> CAN Tx13/2(BDischargeAllowed)  "<BDischargeAllowed>"
  Bus Selector14/9 -> CAN Tx14/11(TMotorRL)  "<TMotorRL>"
  Bus Selector14/4 -> CAN Tx14/6(TInvRL)  "<TInvRL>"
  Bus Selector14/6 -> CAN Tx14/8(TMotorFL)  "<TMotorFL>"
  Bus Selector14/1 -> CAN Tx14/3(TInvFL)  "<TInvFL>"
  Bus Selector14/10 -> CAN Tx14/12(TMotorRR)  "<TMotorRR>"
  Bus Selector14/5 -> CAN Tx14/7(TInvRR)  "<TInvRR>"
  Bus Selector14/7 -> CAN Tx14/9(TMotorFR)  "<TMotorFR>"
  Bus Selector14/2 -> CAN Tx14/4(TInvFR)  "<TInvFR>"
  Bus Selector14/3 -> CAN Tx14/5(TInvMax)  "<TInvMax>"
  Bus Selector14/8 -> CAN Tx14/10(TMotorMax)  "<TMotorMax>"
  Bus Selector15/3 -> CAN Tx15/4(NInvDTCRL)  "<NInvDTCRL>"
  Bus Selector15/1 -> CAN Tx15/2(NInvDTCFL)  "<NInvDTCFL>"
  Bus Selector15/4 -> CAN Tx15/5(NInvDTCRR)  "<NInvDTCRR>"
  Bus Selector15/5 -> CAN Tx15/6(TCellMax)  "<TCellMax>"
  Bus Selector15/6 -> CAN Tx15/7(VCellDelta)  "<VCellDelta>"
  Bus Selector16/7 -> CAN Tx16/8(VCDAccu)  "<VDCAccumulator>"
  Bus Selector16/4 -> CAN Tx16/5(IBMSHallEffect)  "<IBMSHallEffect>"
  Bus Selector16/8 -> CAN Tx16/9(VCDInvRL)  "<VDCInvRL>"
  Bus Selector16/5 -> CAN Tx16/6(IIVTS)  "<IIVTS>"
  Bus Selector16/6 -> CAN Tx16/7(MTotalRequested)  "<MTotalRequested>"
  Bus Selector16/2 -> CAN Tx16/3(BEMSActivated)  "<BEMSActivated>"
  Bus Selector16/3 -> CAN Tx16/4(BTractionControlActivated)  "<BTractionControlActivated>"
  Bus Selector16/1 -> CAN Tx16/2(BAccumulatorFanOn)  "<BAccumulatorFanOn>"
  Bus Selector17/4 -> CAN Tx17/6(VCellMin)  "<VCellMin>"
  Bus Selector17/3 -> CAN Tx17/5(VCellMax)  "<VCellMax>"
  Bus Selector17/2 -> CAN Tx17/3(TCellMin)  "<TCellMin>"
  Bus Selector17/1 -> CAN Tx17/2(NTractionControlKpSelector)  "<NTractionControlKpSelector>"
  Bus Selector18/3 -> CAN Tx18/4(nYawRateErrorActual)  "<nYawRateErrorActual>"
  Bus Selector18/7 -> CAN Tx18/8(tPedalOverlap)  "<tPedalOverlap>"
  Bus Selector18/6 -> CAN Tx18/7(tAppsTimer)  "<tAppsTimer>"
  Bus Selector18/2 -> CAN Tx18/3(aSteeringAngle)  "<aSteeringAngle>"
  Bus Selector18/1 -> CAN Tx18/2(PDischargeLimited)  "<PDischargeLimited>"
  Bus Selector18/5 -> CAN Tx18/6(rSplitRear)  "<rSplitRear>"
  Bus Selector15/2 -> CAN Tx15/3(NInvDTCFR)  "<NInvDTCFR>"
  Bus Selector5/10 -> CAN Tx4/12(rSOC)  "<rSOC>"
  [InverterRRBus] -> CAN1_2Bus/4  "InverterRRCANBus"
  [InverterRLBus] -> CAN1_2Bus/3  "InverterRLCANBus"
  [InverterFRBus] -> CAN1_2Bus/2  "InverterFRCANBus"
  [InverterFLBus] -> CAN1_2Bus/1  "InverterFLCANBus"
  VDamperPotentiometerRL/1 -> Bus Creator1/5  "VDamperPotentiometerRL"
  VDamperPotentiometerRR/1 -> Bus Creator1/6  "VDamperPotentiometerRR"
  Bus Creator19/1 -> [InverterRRBus]
  Multiplexer?/1 -> CAN Tx4/2(Multiplexer05)
  Multiplexer1?/1 -> CAN Tx14/2(Multiplexer15)
  Bus Selector18/4 -> CAN Tx18/5(rRegenPaddle)  "<rRegenPaddle>"
  Bus Selector5/2 -> CAN Tx4/4(NBMSState)  "<NBMSState>"
  [InverterFLBus] -> CAN1_2Bus1/1  "InverterFLCANBus"
  [PDM_Status_3] -> Bus Creator16/8  "PDM_Status_3"
  [DDU7_Analoge_1] -> Bus Creator16/1  "DDU7_Analoge_1"
  [SteeringWheelBus] -> Bus Creator16/12  "SteeringWheelBus"
  [OXTSDataFrame1540] -> Bus Creator16/3  "OXTSDataFrame1540"
  Bus Creator16/1 -> Model1/2
  [PDM_Analoge_2] -> Bus Creator16/10  "PDM_Analoge_2"
  [InverterRLBus] -> CAN1_2Bus1/3  "InverterRLCANBus"
  [PDM_Analoge_3] -> Bus Creator16/11  "PDM_Analoge_3"
  [OXTSDataFrame1541] -> Bus Creator16/4  "OXTSDataFrame1541"
  [DDU7_Analoge_2] -> Bus Creator16/2  "DDU7_Analoge_2"
  CAN1_2Bus1/1 -> Model1/1
  [OXTSDataFrame1544] -> Bus Creator16/5  "OXTSDataFrame1544"
  Model1/1 -> Terminator/1
  [InverterRRBus] -> CAN1_2Bus1/4  "InverterRRCANBus"
  [PDM_Analog_1] -> Bus Creator16/9  "PDM_Analoge_1"
  [InverterFRBus] -> CAN1_2Bus1/2  "InverterFRCANBus"
  [BMSCAN] -> Model1/3
  [PDM_Status_2] -> Bus Creator16/7  "PDM_Status_2"
  [PDM_Status_1] -> Bus Creator16/6  "PDM_Status_1"
  [InverterFLBus] -> CAN1_2Bus2/1  "InverterFLCANBus"
  [PDM_Status_3] -> Bus Creator20/8  "PDM_Status_3"
  [DDU7_Analoge_1] -> Bus Creator20/1  "DDU7_Analoge_1"
  [SteeringWheelBus] -> Bus Creator20/12  "SteeringWheelBus"
  [OXTSDataFrame1540] -> Bus Creator20/3  "OXTSDataFrame1540"
  Bus Creator20/1 -> Model2/2
  [PDM_Analoge_2] -> Bus Creator20/10  "PDM_Analoge_2"
  [InverterRLBus] -> CAN1_2Bus2/3  "InverterRLCANBus"
  [PDM_Analoge_3] -> Bus Creator20/11  "PDM_Analoge_3"
  [OXTSDataFrame1541] -> Bus Creator20/4  "OXTSDataFrame1541"
  [DDU7_Analoge_2] -> Bus Creator20/2  "DDU7_Analoge_2"
  CAN1_2Bus2/1 -> Model2/1
  [OXTSDataFrame1544] -> Bus Creator20/5  "OXTSDataFrame1544"
  Model2/1 -> Terminator1/1
  [InverterRRBus] -> CAN1_2Bus2/4  "InverterRRCANBus"
  [PDM_Analog_1] -> Bus Creator20/9  "PDM_Analoge_1"
  [InverterFRBus] -> CAN1_2Bus2/2  "InverterFRCANBus"
  [BMSCAN] -> Model2/3
  [PDM_Status_2] -> Bus Creator20/7  "PDM_Status_2"
  [PDM_Status_1] -> Bus Creator20/6  "PDM_Status_1"
  NOT4/1 -> CAN Rx/Enable
  Digital Port Read1/1 -> NOT4/1
  CAN Rx/1(pBrakeF) -> Bus Creator1/1
  CAN Rx/2(pBrakeR) -> Bus Creator1/2
  [MCPInitialized] -> CAN Tx/1(MCPInitialized)
  Subsystem/1(MCPInitialized) -> [MCPInitialized]
  CAN Rx/3(DDU7_Analog_2) -> [DDU7_Analoge_2]
  CAN Rx/4(PDM_Analog_01) -> [PDM_Analog_1]
  CAN Rx/5(PDM_Analog_02) -> [PDM_Analoge_2]
  CAN Rx/6(PDM_Analog_03) -> [PDM_Analoge_3]
  CAN Rx/7(PDM_Status_01) -> [PDM_Status_1]
  CAN Rx/8(PDM_Status_02) -> [PDM_Status_2]
  CAN Rx/9(PDM_Status_03) -> [PDM_Status_3]
  CAN Rx/10(SteeringWheel) -> [SteeringWheelBus]
  Bus Selector2/1 -> CAN Tx2/2(rSOETargetError)  "<rSOETargetError>"
  [MCPInitialized] -> CAN Tx10/1(MCPInitialized)
  [MCPInitialized] -> CAN Tx13/1(MCPInitialized)
  Bus Selector17/5 -> CAN Tx17/7(VLVSystem)  "<VLVSystem>"
  Constant1/1 -> CAN Tx17/8(tEtasOn)
  Constant/1 -> CAN Tx17/4(TEtas)
  [MCPInitialized] -> CAN Tx3/1(MCPInitialized)
  [MCPInitialized] -> CAN Tx15/1(MCPInitialized)
  [MCPInitialized] -> CAN Tx2/1(MCPInitialized)
  [MCPInitialized] -> CAN Tx14/1(MCPInitialized)
  [MCPInitialized] -> CAN Tx9/1(MCPInitialized)
  [MCPInitialized] -> CAN Tx4/1(MCPInitialized)
  [MCPInitialized] -> CAN Tx1/1(MCPInitialized)
  [MCPInitialized] -> CAN Tx8/1(MCPInitialized)
  [MCPInitialized] -> CAN Tx19/1(MCPInitialized)
  [MCPInitialized] -> CAN Tx17/1(MCPInitialized)
  [MCPInitialized] -> CAN Tx18/1(MCPInitialized)
  [MCPInitialized] -> CAN Tx12/1(MCPInitialized)
  [MCPInitialized] -> CAN Tx5/1(MCPInitialized)
  [MCPInitialized] -> CAN Tx6/1(MCPInitialized)
  [MCPInitialized] -> CAN Tx7/1(MCPInitialized)
  [MCPInitialized] -> CAN Tx11/1(MCPInitialized)
  [MCPInitialized] -> CAN Tx16/1(MCPInitialized)
